simulink model "test_sim2"  (R2019a)
settings: Solver=VariableStepAuto  StartTime=0.0  StopTime=100  RelTol=1e-3
undefined symbols (not defined in the file or in its folder): des_quad10, des_quad20, des_quad30
settings Model: Creator=UFRST25  LastModifiedBy=Rayane
settings DataIOCC: ReturnWorkspaceOutputs=off
settings DebuggingCC: ArithmeticOperatorsInVariantConditions=warning

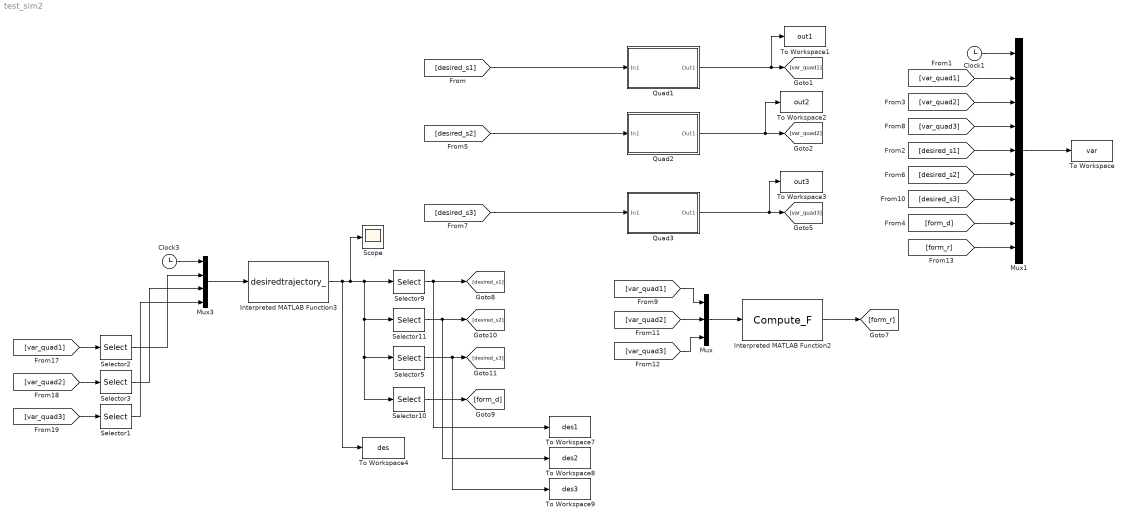
== system test_sim2 ==
  Clock1 : Clock
  Clock3 : Clock
  Interpreted MATLAB Function2 : MATLABFcn  MATLABFcn=Compute_F
  Interpreted MATLAB Function3 : MATLABFcn  MATLABFcn=desiredtrajectory_
  Mux : Mux  Inputs=3
  Mux1 : Mux  Inputs=9
  Mux3 : Mux
  Quad1 : Subsystem
  Quad2 : Subsystem
  Quad3 : Subsystem
  Scope : Scope
  Selector1 : Selector  InputPortWidth=27  IndexOptions=Index vector (dialog)  Indices=[1:3]  OutputSizes=1
  Selector10 : Selector  InputPortWidth=38  IndexOptions=Index vector (dialog)  Indices=[30:38]  OutputSizes=1
  Selector11 : Selector  InputPortWidth=38  IndexOptions=Index vector (dialog)  Indices=[10:18, 28, 29]  OutputSizes=1
  Selector2 : Selector  InputPortWidth=27  IndexOptions=Index vector (dialog)  Indices=[1:3]  OutputSizes=1
  Selector3 : Selector  InputPortWidth=27  IndexOptions=Index vector (dialog)  Indices=[1:3]  OutputSizes=1
  Selector5 : Selector  InputPortWidth=38  IndexOptions=Index vector (dialog)  Indices=[19:27, 28, 29]  OutputSizes=1
  Selector9 : Selector  InputPortWidth=38  IndexOptions=Index vector (dialog)  Indices=[1:9, 28, 29]  OutputSizes=1
  To Workspace : ToWorkspace  VariableName=var  SampleTime=-1
  To Workspace1 : ToWorkspace  VariableName=out1  SampleTime=-1
  To Workspace2 : ToWorkspace  VariableName=out2  SampleTime=-1
  To Workspace3 : ToWorkspace  VariableName=out3  SampleTime=-1
  To Workspace4 : ToWorkspace  VariableName=des  SampleTime=-1
  To Workspace7 : ToWorkspace  VariableName=des1  SampleTime=-1
  To Workspace8 : ToWorkspace  VariableName=des2  SampleTime=-1
  To Workspace9 : ToWorkspace  VariableName=des3  SampleTime=-1
  wires:
  Clock1/1 -> Mux1/1
  [var_quad1] -> Mux1/2
  [desired_s1] -> Mux1/5
  Mux1/1 -> To Workspace/1
  Quad1/1(Out1) -> To Workspace1/1, [var_quad1]
  [desired_s1] -> Quad1/1(In1)
  Quad2/1(Out1) -> To Workspace2/1, [var_quad2]
  [var_quad2] -> Mux1/3
  [form_d] -> Mux1/8
  [desired_s2] -> Quad2/1(In1)
  [desired_s2] -> Mux1/6
  [desired_s3] -> Quad3/1(In1)
  Quad3/1(Out1) -> To Workspace3/1, [var_quad3]
  [var_quad3] -> Mux1/4
  [desired_s3] -> Mux1/7
  [var_quad1] -> Mux/1
  [var_quad2] -> Mux/2
  [var_quad3] -> Mux/3
  Mux/1 -> Interpreted MATLAB Function2/1
  Interpreted MATLAB Function2/1 -> [form_r]
  [form_r] -> Mux1/9
  Interpreted MATLAB Function3/1 -> To Workspace4/1, Scope/1, Selector9/1, Selector10/1, Selector5/1, Selector11/1
  Selector5/1 -> [desired_s3], To Workspace9/1
  Selector11/1 -> [desired_s2], To Workspace8/1
  Selector10/1 -> [form_d]
  Selector9/1 -> [desired_s1], To Workspace7/1
  Mux3/1 -> Interpreted MATLAB Function3/1
  [var_quad2] -> Selector3/1
  Selector2/1 -> Mux3/2
  [var_quad1] -> Selector2/1
  Selector1/1 -> Mux3/4
  Selector3/1 -> Mux3/3
  [var_quad3] -> Selector1/1
  Clock3/1 -> Mux3/1

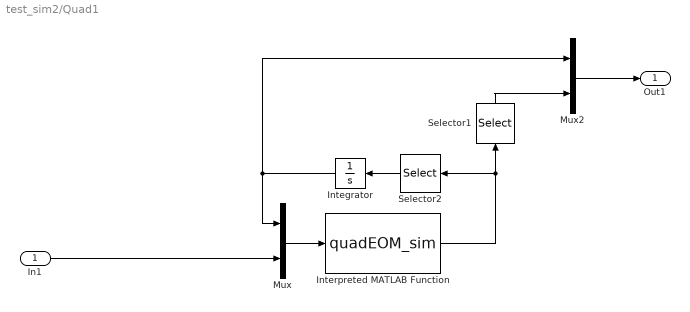
== system test_sim2/Quad1 ==
  In1 : Inport
  Integrator : Integrator  InitialCondition=des_quad10
  Interpreted MATLAB Function : MATLABFcn  MATLABFcn=quadEOM_sim  OutputDimensions=27
  Mux : Mux  Inputs=2
  Mux2 : Mux  Inputs=2
  Selector1 : Selector  InputPortWidth=27  IndexOptions=Index vector (dialog)  Indices=[14:27]  OutputSizes=1
  Selector2 : Selector  InputPortWidth=27  IndexOptions=Index vector (dialog)  Indices=[1:13]  OutputSizes=1
  Out1 : Outport
  wires:
  In1/1 -> Mux/2
  Selector2/1 -> Integrator/1
  Integrator/1 -> Mux2/1, Mux/1
  Interpreted MATLAB Function/1 -> Selector2/1, Selector1/1
  Selector1/1 -> Mux2/2
  Mux/1 -> Interpreted MATLAB Function/1
  Mux2/1 -> Out1/1

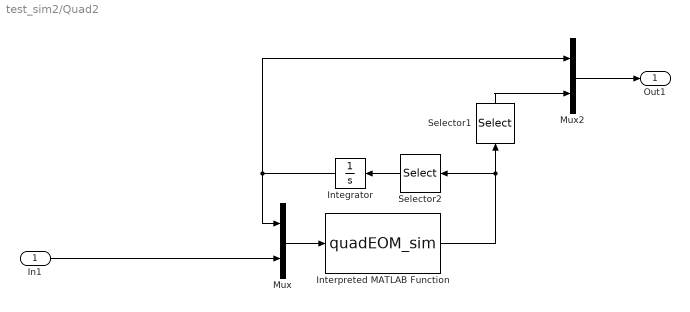
== system test_sim2/Quad2 ==
  In1 : Inport
  Integrator : Integrator  InitialCondition=des_quad20
  Interpreted MATLAB Function : MATLABFcn  MATLABFcn=quadEOM_sim  OutputDimensions=27
  Mux : Mux  Inputs=2
  Mux2 : Mux  Inputs=2
  Selector1 : Selector  InputPortWidth=27  IndexOptions=Index vector (dialog)  Indices=[14:27]  OutputSizes=1
  Selector2 : Selector  InputPortWidth=27  IndexOptions=Index vector (dialog)  Indices=[1:13]  OutputSizes=1
  Out1 : Outport
  wires:
  Mux2/1 -> Out1/1
  Mux/1 -> Interpreted MATLAB Function/1
  Selector1/1 -> Mux2/2
  Interpreted MATLAB Function/1 -> Selector1/1, Selector2/1
  Integrator/1 -> Mux/1, Mux2/1
  Selector2/1 -> Integrator/1
  In1/1 -> Mux/2

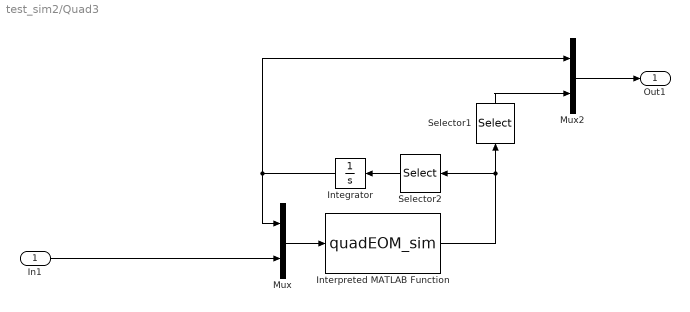
== system test_sim2/Quad3 ==
  In1 : Inport
  Integrator : Integrator  InitialCondition=des_quad30
  Interpreted MATLAB Function : MATLABFcn  MATLABFcn=quadEOM_sim  OutputDimensions=27
  Mux : Mux  Inputs=2
  Mux2 : Mux  Inputs=2
  Selector1 : Selector  InputPortWidth=27  IndexOptions=Index vector (dialog)  Indices=[14:27]  OutputSizes=1
  Selector2 : Selector  InputPortWidth=27  IndexOptions=Index vector (dialog)  Indices=[1:13]  OutputSizes=1
  Out1 : Outport
  wires:
  In1/1 -> Mux/2
  Selector2/1 -> Integrator/1
  Integrator/1 -> Mux2/1, Mux/1
  Interpreted MATLAB Function/1 -> Selector2/1, Selector1/1
  Selector1/1 -> Mux2/2
  Mux/1 -> Interpreted MATLAB Function/1
  Mux2/1 -> Out1/1
